simulink model "Model_Following_Destrete"  (Simulink 8.5)
settings: Solver=ode45  StartTime=0.0  StopTime=10.0  RelTol=1e-3
values from neighbouring files (symbols this model uses):
  A = [10 0 0 0 0 0 0 0 0 0 0 20 ... (100 elements, 10x10)]    [ABC.mat]    (also in AMB_5DOF_Destrete.m = [])
  B = [0.0298026407502 0.626638455375 0.592170443728 0.0619918589601 0.174230290231 0.098145354036 0.7829204017 0.517538751148 0.138142473448 0.16685524493 0.812558669985 0.867388222232 ... (50 elements, 10x5)]    [ABC.mat]    (also in AMB_5DOF_Destrete.m = [])
  C = [0.0803132148797 0.588234790038 0.200871010197 0.657679571025 0.0466720902179 0.469816709225 0.246091528714 0.78856831003 0.741681028429 0.942191544436 0.593515897954 0.194588427722 ... (50 elements, 5x10)]    [ABC.mat]    (also in AMB_5DOF_Destrete.m = [])
  Cd = inv(Rd_wave)*H'*(inv((G-H*Kd)'-eye(nr))*(G-H*Kd)'-eye(nr))*P*gd    [AMB_5DOF_Destrete.m]
  Cu_star = inv(Rd_wave)*(H'*inv((G-H*Kd)'-eye(nr))*Kd'+eye(mr))*Rd    [AMB_5DOF_Destrete.m]
  D = zeros(pr,mr)    [AMB_5DOF_Destrete.m]
  Ed = inv(Rd_wave)*(D'+H'*inv(eye(nr)-(G-H*Kd)')*(C-D*Kd)')*Qd    [AMB_5DOF_Destrete.m]
  Ts = 2.5e-4    (= 0.00025)    [AMB_5DOF_Destrete.m]
  ud_star = [0 0 0 0 0]'    [AMB_5DOF_Destrete.m]
undefined symbols (not defined in the file or in its folder): Kd, x
settings Model: Creator=koni  LastModifiedBy=123
settings DebuggingCC: SolverPrmCheckMsg=warning  FcnCallInpInsideContextMsg=UseLocalSettings

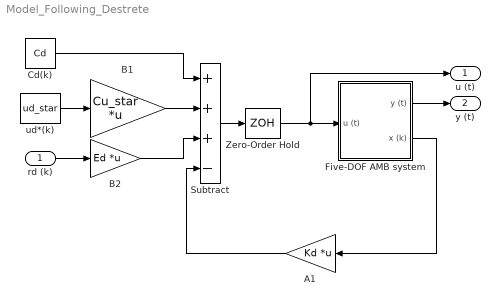
== system Model_Following_Destrete ==
  rd (k) : Inport  PortDimensions=pr
  " Five-DOF AMB system" : Subsystem
  A1 : Gain  Gain=Kd  Multiplication=Matrix(K*u)
  B1 : Gain  Gain=Cu_star  Multiplication=Matrix(K*u)
  B2 : Gain  Gain=Ed  Multiplication=Matrix(K*u)
  Cd(k) : Constant  Value=Cd
  Subtract : Sum  Inputs=+++-
  Zero-Order Hold : ZeroOrderHold  SampleTime=Ts
  ud*(k) : Constant  Value=ud_star
  u (t) : Outport  PortDimensions=mr
  y (t) : Outport  Port=2  PortDimensions=pr
  wires:
  " Five-DOF AMB system"/1(y (t)) -> y (t)/1
  Subtract/1 -> Zero-Order Hold/1
  B2/1 -> Subtract/3
  rd (k)/1 -> B2/1
  " Five-DOF AMB system"/2(x (k)) -> A1/1
  A1/1 -> Subtract/4
  ud*(k)/1 -> B1/1
  B1/1 -> Subtract/2
  Cd(k)/1 -> Subtract/1
  Zero-Order Hold/1 -> " Five-DOF AMB system"/1(u (t)), u (t)/1

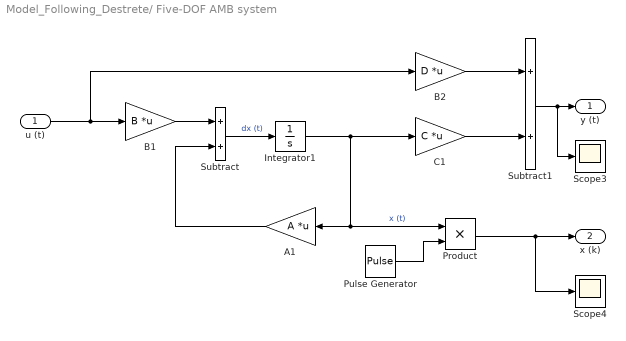
== system Model_Following_Destrete/ Five-DOF AMB system ==
  u (t) : Inport  PortDimensions=mr
  A1 : Gain  Gain=A  Multiplication=Matrix(K*u)
  B1 : Gain  Gain=B  Multiplication=Matrix(K*u)
  B2 : Gain  Gain=D  Multiplication=Matrix(K*u)
  C1 : Gain  Gain=C  Multiplication=Matrix(K*u)
  Integrator1 : Integrator  InitialCondition=x(:,1)
  Product : Product
  Pulse Generator : DiscretePulseGenerator  PulseType=Time based  Period=Ts
  Scope3 : Scope
      settings: TimeRange=0.05  SaveName=ScopeData2
  Scope4 : Scope
      settings: TimeRange=0.04999  YMin=-0.001  YMax=0.006  SaveName=ScopeData3
  Subtract : Sum
  Subtract1 : Sum
  y (t) : Outport  PortDimensions=pr
  x (k) : Outport  Port=2  PortDimensions=nr
  wires:
  Subtract/1 -> Integrator1/1  "dx (t)"
  Integrator1/1 -> C1/1, A1/1, Product/1  "x (t)"
  u (t)/1 -> B1/1, B2/1
  B1/1 -> Subtract/1
  A1/1 -> Subtract/2
  Subtract1/1 -> Scope3/1, y (t)/1
  C1/1 -> Subtract1/2
  B2/1 -> Subtract1/1
  Product/1 -> Scope4/1, x (k)/1
  Pulse Generator/1 -> Product/2
